simulink model "Test"  (R2021b)
settings: Solver=VariableStepAuto  StartTime=0.0  StopTime=10.0  RelTol=1e-3
undefined symbols (not defined in the file): id, IOSIG_AI_FUEL_IN, NVM_CFG_VEHCLE_MODEL, rte_set_uint8_val, RXSIG_CPD1_FuelMassSignal, SIG_CLASS_COMRX, SIG_CLASS_COMTX, SIG_CLASS_HMI_SND, SIG_CLASS_HMI_TT, SIG_CLASS_IOAL, SIG_CLASS_NVM_CFG, SIG_CLASS_SWC, SIG_CLASS_SYS, SND_FUEL_LEVEL_LOW, SYSSIG_LNN_MODE, SYSSIG_TICK_COUNT, TNC_FuelPrcDisp, TNC_FuelPrcReal, TT_FUEL_LEVEL_LOW, TXSIG_MD_OilPercent, type, val, VEL_VehicleRealSpeed
libraries: simulink x1
(part 1 of 2)
settings Model: Creator=黄艳龙  LastModifiedBy=黄艳龙

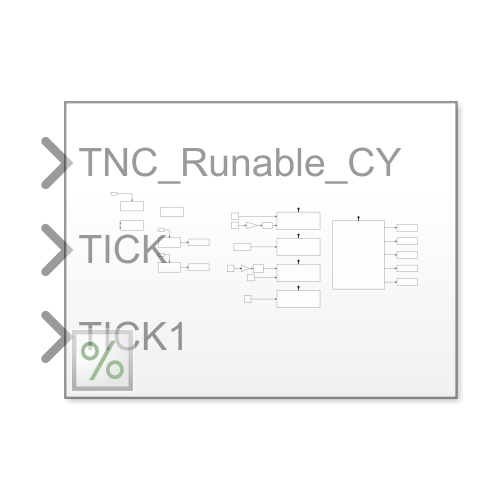
[thumbnail: Simulink's stored preview of the top-level diagram]
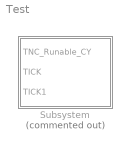
== system Test ==
  Subsystem : Subsystem  Commented=on

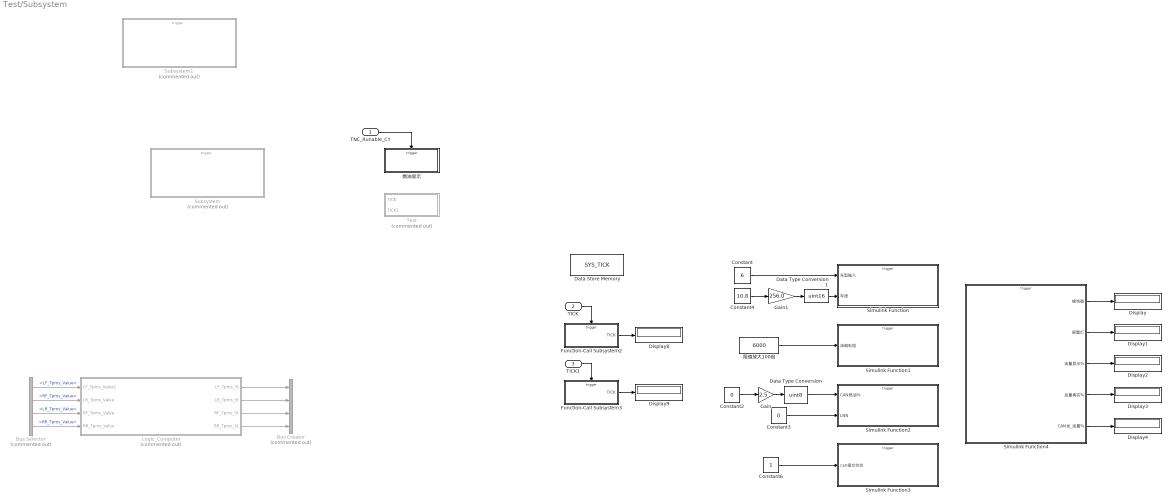
== system Test/Subsystem ==
  TNC_Runable_CY : Inport  SampleTime=1  OutputFunctionCall=on
  TICK : Inport  Priority=1  Port=2  SampleTime=0.001  OutputFunctionCall=on
  TICK1 : Inport  Priority=1  Port=3  SampleTime=0.001  OutputFunctionCall=on
  Bus Creator : BusCreator  Commented=on  Inputs=4
  Bus Selector : BusSelector  Commented=on  OutputSignals=LF_Tpms_Value,RF_Tpms_Value,LR_Tpms_Value,RR_Tpms_Value
  Constant : Constant  Value=6  OutDataTypeStr=uint16
  Constant2 : Constant  Value=0  OutDataTypeStr=single
  Constant3 : Constant  Value=0  OutDataTypeStr=uint8
  Constant4 : Constant  Value=10.8  OutDataTypeStr=single
  Constant6 : Constant  OutDataTypeStr=uint8
  Data Store Memory : DataStoreMemory  DataStoreName=SYS_TICK  ReadBeforeWriteMsg=warning  WriteAfterWriteMsg=warning  WriteAfterReadMsg=warning  ShowAdditionalParam=off  OutDataTypeStr=uint32
  Data Type Conversion : DataTypeConversion  OutDataTypeStr=uint8  RndMeth=Round
  Data Type Conversion1 : DataTypeConversion  OutDataTypeStr=uint16  RndMeth=Round
  Display{,1..4,8..9} (7 alike) : Display
      settings: Format=decimal (Stored Integer)
  Function-Call Subsystem2 : Subsystem  TreatAsAtomicUnit=on
  Function-Call Subsystem3 : Subsystem  TreatAsAtomicUnit=on
  Gain : Gain  Gain=2.5  ParamDataTypeStr=single  OutDataTypeStr=uint8  RndMeth=Round
  Gain1 : Gain  Gain=256.0  ParamDataTypeStr=single  OutDataTypeStr=single
  Logic_Computer : Subsystem  Commented=on
  Simulink Function : Subsystem  TreatAsAtomicUnit=on
  Simulink Function1 : Subsystem  TreatAsAtomicUnit=on
  Simulink Function2 : Subsystem  TreatAsAtomicUnit=on
  Simulink Function3 : Subsystem  TreatAsAtomicUnit=on
  Simulink Function4 : Subsystem  TreatAsAtomicUnit=on
  Subsystem : Subsystem  Commented=on
  Subsystem1 : Subsystem  Commented=on
  Test : Subsystem  Commented=on
  燃油显示 : Subsystem  TreatAsAtomicUnit=on
  阻值放大100倍 : Constant  Value=6000  OutDataTypeStr=uint32
  wires:
  Data Type Conversion1/1 -> Simulink Function/2(车速)
  Constant/1 -> Simulink Function/1(车型输入)
  Gain/1 -> Data Type Conversion/1
  Simulink Function4/1(蜂鸣器) -> Display/1
  Gain1/1 -> Data Type Conversion1/1
  TICK/1 -> Function-Call Subsystem2/Trigger
  Simulink Function4/5(CAN发_油量%) -> Display4/1
  Function-Call Subsystem2/1(TICK) -> Display8/1
  Simulink Function4/3(油量显示%) -> Display2/1
  阻值放大100倍/1 -> Simulink Function1/1(油箱电阻)
  Simulink Function4/4(油量真实%) -> Display3/1
  Data Type Conversion/1 -> Simulink Function2/1(CAN燃油%)
  Constant4/1 -> Gain1/1
  Constant6/1 -> Simulink Function3/1(can报文状态)
  Simulink Function4/2(报警灯) -> Display1/1
  Constant3/1 -> Simulink Function2/2(LNN)
  TICK1/1 -> Function-Call Subsystem3/Trigger
  Function-Call Subsystem3/1(TICK) -> Display9/1
  Constant2/1 -> Gain/1
  TNC_Runable_CY/1 -> 燃油显示/Trigger
  Bus Selector/3 -> Logic_Computer/3(RF_Tpms_Value)  "<LR_Tpms_Value>"
  Logic_Computer/1(LF_Tpms_St) -> Bus Creator/1
  Logic_Computer/2(LR_Tpms_St) -> Bus Creator/2
  Bus Selector/2 -> Logic_Computer/2(LR_Tpms_Value)  "<RF_Tpms_Value>"
  Bus Selector/4 -> Logic_Computer/4(RR_Tpms_Value)  "<RR_Tpms_Value>"
  Bus Selector/1 -> Logic_Computer/1(LF_Tpms_Value1)  "<LF_Tpms_Value>"
  Logic_Computer/3(RF_Tpms_St) -> Bus Creator/3
  Logic_Computer/4(RR_Tpms_St) -> Bus Creator/4

== system Test/Subsystem/Function-Call Subsystem2 ==
  function : TriggerPort  TriggerType=function-call  VariantControl=(inherit)
  Add : Sum
  Constant : Constant  OutDataTypeStr=uint32
  Data Store Read : DataStoreRead  DataStoreName=SYS_TICK  IndexOptions=Index vector (dialog)  Indices=1  OutputSizes=1
  Data Store Write : DataStoreWrite  DataStoreName=SYS_TICK  IndexOptions=Index vector (dialog)  Indices=1  OutputSizes=1
  TICK : Outport  OutDataTypeStr=uint32
  wires:
  Data Store Read/1 -> Add/1
  Add/1 -> TICK/1, Data Store Write/1
  Constant/1 -> Add/2

== system Test/Subsystem/Function-Call Subsystem3 ==
  function : TriggerPort  TriggerType=function-call  VariantControl=(inherit)
  Add : Sum
  Constant : Constant  OutDataTypeStr=uint32
  Data Store Write : DataStoreWrite  Commented=on  DataStoreName=SYS_TICK  IndexOptions=Index vector (dialog)  Indices=1  OutputSizes=1
  Unit Delay : UnitDelay  SampleTime=-1  HasFrameUpgradeWarning=on
  TICK : Outport  OutDataTypeStr=uint32
  wires:
  Add/1 -> Data Store Write/1, Unit Delay/1, TICK/1
  Constant/1 -> Add/1
  Unit Delay/1 -> Add/2

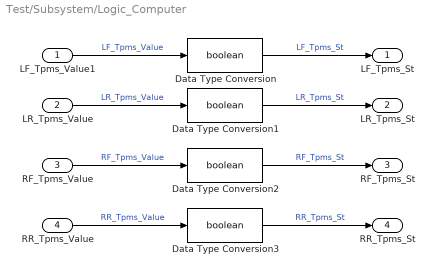
== system Test/Subsystem/Logic_Computer ==
  LF_Tpms_Value1 : Inport
  LR_Tpms_Value : Inport  Port=2
  RF_Tpms_Value : Inport  Port=3
  RR_Tpms_Value : Inport  Port=4
  Data Type Conversion{,1..3} (4 alike) : DataTypeConversion  OutDataTypeStr=boolean
  LF_Tpms_St : Outport
  LR_Tpms_St : Outport  Port=2
  RF_Tpms_St : Outport  Port=3
  RR_Tpms_St : Outport  Port=4
  wires:
  RR_Tpms_Value/1 -> Data Type Conversion3/1  "RR_Tpms_Value"
  RF_Tpms_Value/1 -> Data Type Conversion2/1  "RF_Tpms_Value"
  LR_Tpms_Value/1 -> Data Type Conversion1/1  "LR_Tpms_Value"
  LF_Tpms_Value1/1 -> Data Type Conversion/1  "LF_Tpms_Value"
  Data Type Conversion/1 -> LF_Tpms_St/1  "LF_Tpms_St"
  Data Type Conversion1/1 -> LR_Tpms_St/1  "LR_Tpms_St"
  Data Type Conversion2/1 -> RF_Tpms_St/1  "RF_Tpms_St"
  Data Type Conversion3/1 -> RR_Tpms_St/1  "RR_Tpms_St"

== system Test/Subsystem/Simulink Function ==
  车型输入 : Inport  OutDataTypeStr=uint16
  车速 : Inport  Port=2  OutDataTypeStr=uint16
  rte_get_uint16_val : TriggerPort  TriggerType=function-call  IsSimulinkFunction=on  FunctionName=rte_get_uint16_val  FunctionVisibility=scoped  VariantControl=(inherit)
  If : If  IfExpression=u1==21  ElseIfExpressions=u1==18  ShowElse=off
  Merge : Merge
  Terminator : Terminator
  车型_ : Subsystem  TreatAsAtomicUnit=on
  车速_ : Subsystem  TreatAsAtomicUnit=on
  type : ArgIn  DisableCoverage=on  OutDataTypeStr=uint8  ArgumentName=type
  id : ArgIn  DisableCoverage=on  Port=2  OutDataTypeStr=uint16  ArgumentName=id
  val : ArgOut  DisableCoverage=on  OutDataTypeStr=uint16  ArgumentName=val
  wires:
  type/1 -> Terminator/1
  id/1 -> If/1
  If/1 -> 车型_/Action
  If/2 -> 车速_/Action
  车型_/1(Out1) -> Merge/1
  车速_/1(Out1) -> Merge/2
  Merge/1 -> val/1
  车型输入/1 -> 车型_/1(车型输入)
  车速/1 -> 车速_/1(车型输入1)

== system Test/Subsystem/Simulink Function1 ==
  油箱电阻 : Inport  OutDataTypeStr=uint32
  rte_get_uint32_val : TriggerPort  TriggerType=function-call  IsSimulinkFunction=on  FunctionName=rte_get_uint32_val  FunctionVisibility=scoped  VariantControl=(inherit)
  Data Store Read : DataStoreRead  DataStoreName=SYS_TICK  IndexOptions=Index vector (dialog)  Indices=1  OutputSizes=1
  If : If  IfExpression=u1==17  ElseIfExpressions=u1==14  ShowElse=off
  If Action Subsystem : Subsystem  TreatAsAtomicUnit=on
  If Action Subsystem1 : Subsystem  TreatAsAtomicUnit=on
  Merge : Merge
  Terminator : Terminator
  type : ArgIn  DisableCoverage=on  OutDataTypeStr=uint8  ArgumentName=type
  id : ArgIn  DisableCoverage=on  Port=2  OutDataTypeStr=uint16  ArgumentName=id
  val : ArgOut  DisableCoverage=on  OutDataTypeStr=uint32  ArgumentName=val
  wires:
  type/1 -> Terminator/1
  id/1 -> If/1
  Merge/1 -> val/1
  If/1 -> If Action Subsystem/Action
  油箱电阻/1 -> If Action Subsystem/1(油箱电阻)
  Data Store Read/1 -> If Action Subsystem1/1(时间)
  If/2 -> If Action Subsystem1/Action
  If Action Subsystem/1(Out1) -> Merge/1
  If Action Subsystem1/1(Out1) -> Merge/2

== system Test/Subsystem/Simulink Function2 ==
  CAN燃油% : Inport  OutDataTypeStr=uint8
  LNN : Inport  Port=2  OutDataTypeStr=uint8
  rte_get_uint8_val : TriggerPort  TriggerType=function-call  IsSimulinkFunction=on  FunctionName=rte_get_uint8_val  FunctionVisibility=scoped  VariantControl=(inherit)
  Merge : Merge
  Switch Case : SwitchCase  CaseConditions={15,13}
  Terminator : Terminator
  Terminator1 : Terminator
  _ : Subsystem  TreatAsAtomicUnit=on
  车速_ : Subsystem  TreatAsAtomicUnit=on
  u : ArgIn  DisableCoverage=on  OutDataTypeStr=uint8  ArgumentName=type
  u1 : ArgIn  DisableCoverage=on  Port=2  OutDataTypeStr=uint16  ArgumentName=id
  y : ArgOut  DisableCoverage=on  OutDataTypeStr=uint8  ArgumentName=val
  wires:
  u/1 -> Terminator/1
  u1/1 -> Switch Case/1
  Switch Case/1 -> _/Action
  _/1(Out1) -> Merge/1
  车速_/1(Out1) -> Merge/2
  Merge/1 -> y/1
  CAN燃油%/1 -> _/1(in)
  LNN/1 -> 车速_/1(in)
  Switch Case/2 -> 车速_/Action
  Switch Case/3 -> Terminator1/1

== system Test/Subsystem/Simulink Function3 ==
  can报文状态 : Inport  OutDataTypeStr=uint8
  rte_com_get_rxsig_state : TriggerPort  TriggerType=function-call  IsSimulinkFunction=on  FunctionName=rte_com_get_rxsig_state  FunctionVisibility=scoped  VariantControl=(inherit)
  Terminator1 : Terminator
  id : ArgIn  DisableCoverage=on  OutDataTypeStr=uint16  ArgumentName=id
  val : ArgOut  DisableCoverage=on  OutDataTypeStr=uint8  ArgumentName=val
  wires:
  id/1 -> Terminator1/1
  can报文状态/1 -> val/1

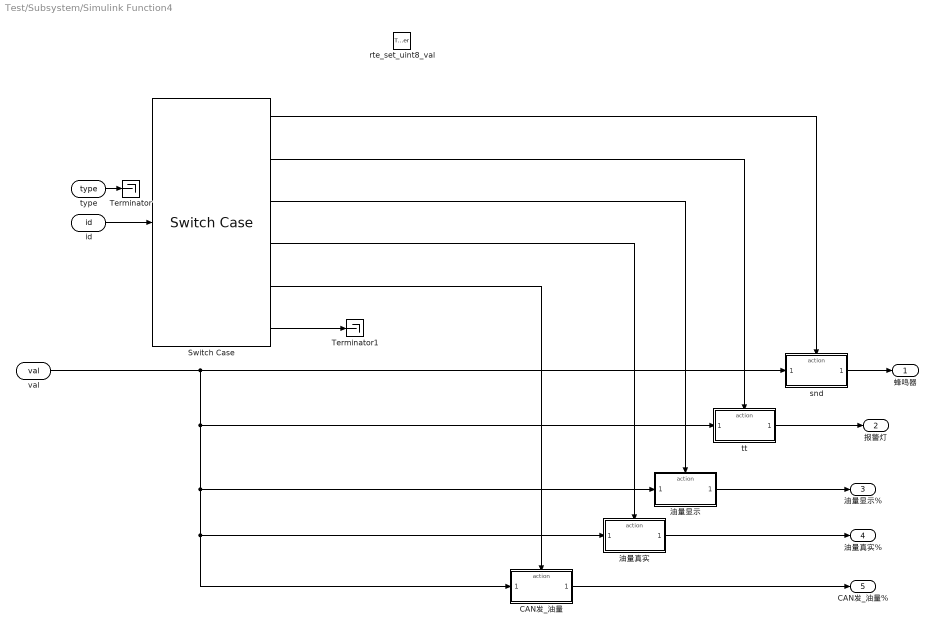
== system Test/Subsystem/Simulink Function4 ==
  rte_set_uint8_val : TriggerPort  TriggerType=function-call  IsSimulinkFunction=on  FunctionName=rte_set_uint8_val  FunctionVisibility=scoped  VariantControl=(inherit)
  CAN发_油量 : Subsystem  TreatAsAtomicUnit=on
  Switch Case : SwitchCase  CaseConditions={23,22,19,20,16}
  Terminator : Terminator
  Terminator1 : Terminator
  snd : Subsystem  TreatAsAtomicUnit=on
  tt : Subsystem  TreatAsAtomicUnit=on
  油量显示 : Subsystem  TreatAsAtomicUnit=on
  油量真实 : Subsystem  TreatAsAtomicUnit=on
  type : ArgIn  DisableCoverage=on  OutDataTypeStr=uint8  ArgumentName=type
  id : ArgIn  DisableCoverage=on  Port=2  OutDataTypeStr=uint16  ArgumentName=id
  val : ArgIn  DisableCoverage=on  Port=3  OutDataTypeStr=uint8  ArgumentName=val
  蜂鸣器 : Outport  OutDataTypeStr=uint8
  报警灯 : Outport  Port=2  OutDataTypeStr=uint8
  油量显示% : Outport  Port=3  OutDataTypeStr=uint8
  油量真实% : Outport  Port=4  OutDataTypeStr=uint8
  CAN发_油量% : Outport  Port=5  OutDataTypeStr=uint8
  wires:
  type/1 -> Terminator/1
  id/1 -> Switch Case/1
  snd/1(Output) -> 蜂鸣器/1
  tt/1(Output1) -> 报警灯/1
  Switch Case/1 -> snd/Action
  Switch Case/2 -> tt/Action
  Switch Case/3 -> 油量显示/Action
  油量显示/1(Output1) -> 油量显示%/1
  Switch Case/4 -> 油量真实/Action
  油量真实/1(Output1) -> 油量真实%/1
  Switch Case/5 -> CAN发_油量/Action
  CAN发_油量/1(Output1) -> CAN发_油量%/1
  val/1 -> snd/1(车型输入), tt/1(车型输入), CAN发_油量/1(车型输入), 油量真实/1(车型输入), 油量显示/1(车型输入)
  Switch Case/6 -> Terminator1/1

== system Test/Subsystem/Subsystem ==
  function : TriggerPort  TriggerType=function-call  VariantControl=(inherit)
  Constant : Constant
  Constant1 : Constant
  Function Caller : FunctionCaller  FunctionPrototype=val = rte_get_uint8_val(x,y)  InputArgumentSpecifications=<Enter example>  OutputArgumentSpecifications=<Enter example>
  Scope : Scope
  Simulink Function : Subsystem  TreatAsAtomicUnit=on
  wires:
  Constant/1 -> Function Caller/1
  Constant1/1 -> Function Caller/2
  Function Caller/1 -> Scope/1

== system Test/Subsystem/Subsystem1 ==
  function : TriggerPort  TriggerType=function-call  VariantControl=(inherit)
  Constant : Constant
  Constant1 : Constant
  Function Caller : FunctionCaller  FunctionPrototype=val = rte_get_uint8_val(x,y)  InputArgumentSpecifications=<Enter example>  OutputArgumentSpecifications=<Enter example>
  Scope : Scope
  Simulink Function : Subsystem  TreatAsAtomicUnit=on
  wires:
  Constant/1 -> Function Caller/1
  Constant1/1 -> Function Caller/2
  Function Caller/1 -> Scope/1

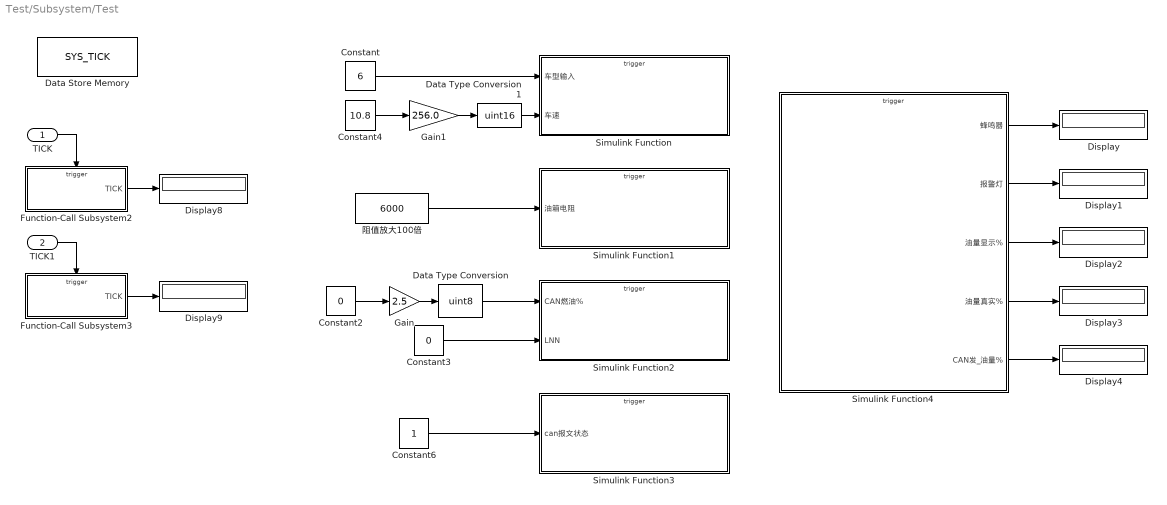
== system Test/Subsystem/Test ==
  TICK : Inport  Priority=1  SampleTime=0.001  OutputFunctionCall=on
  TICK1 : Inport  Priority=1  Port=2  SampleTime=0.001  OutputFunctionCall=on
  Constant : Constant  Value=6  OutDataTypeStr=uint16
  Constant2 : Constant  Value=0  OutDataTypeStr=single
  Constant3 : Constant  Value=0  OutDataTypeStr=uint8
  Constant4 : Constant  Value=10.8  OutDataTypeStr=single
  Constant6 : Constant  OutDataTypeStr=uint8
  Data Store Memory : DataStoreMemory  DataStoreName=SYS_TICK  ReadBeforeWriteMsg=warning  WriteAfterWriteMsg=warning  WriteAfterReadMsg=warning  ShowAdditionalParam=off  OutDataTypeStr=uint32
  Data Type Conversion : DataTypeConversion  OutDataTypeStr=uint8  RndMeth=Round
  Data Type Conversion1 : DataTypeConversion  OutDataTypeStr=uint16  RndMeth=Round
  Display{,1..4,8..9} (7 alike) : Display
      settings: Format=decimal (Stored Integer)
  Function-Call Subsystem2 : Subsystem  TreatAsAtomicUnit=on
  Function-Call Subsystem3 : Subsystem  TreatAsAtomicUnit=on
  Gain : Gain  Gain=2.5  ParamDataTypeStr=single  OutDataTypeStr=uint8  RndMeth=Round
  Gain1 : Gain  Gain=256.0  ParamDataTypeStr=single  OutDataTypeStr=single
  Simulink Function : Subsystem  TreatAsAtomicUnit=on
  Simulink Function1 : Subsystem  TreatAsAtomicUnit=on
  Simulink Function2 : Subsystem  TreatAsAtomicUnit=on
  Simulink Function3 : Subsystem  TreatAsAtomicUnit=on
  Simulink Function4 : Subsystem  TreatAsAtomicUnit=on
  阻值放大100倍 : Constant  Value=6000  OutDataTypeStr=uint32
  wires:
  Constant/1 -> Simulink Function/1(车型输入)
  Simulink Function4/3(油量显示%) -> Display2/1
  Simulink Function4/2(报警灯) -> Display1/1
  Function-Call Subsystem3/1(TICK) -> Display9/1
  Simulink Function4/5(CAN发_油量%) -> Display4/1
  Constant4/1 -> Gain1/1
  Simulink Function4/4(油量真实%) -> Display3/1
  Constant6/1 -> Simulink Function3/1(can报文状态)
  Constant3/1 -> Simulink Function2/2(LNN)
  Constant2/1 -> Gain/1
  Gain/1 -> Data Type Conversion/1
  TICK/1 -> Function-Call Subsystem2/Trigger
  Function-Call Subsystem2/1(TICK) -> Display8/1
  阻值放大100倍/1 -> Simulink Function1/1(油箱电阻)
  Data Type Conversion1/1 -> Simulink Function/2(车速)
  Gain1/1 -> Data Type Conversion1/1
  TICK1/1 -> Function-Call Subsystem3/Trigger
  Simulink Function4/1(蜂鸣器) -> Display/1
  Data Type Conversion/1 -> Simulink Function2/1(CAN燃油%)

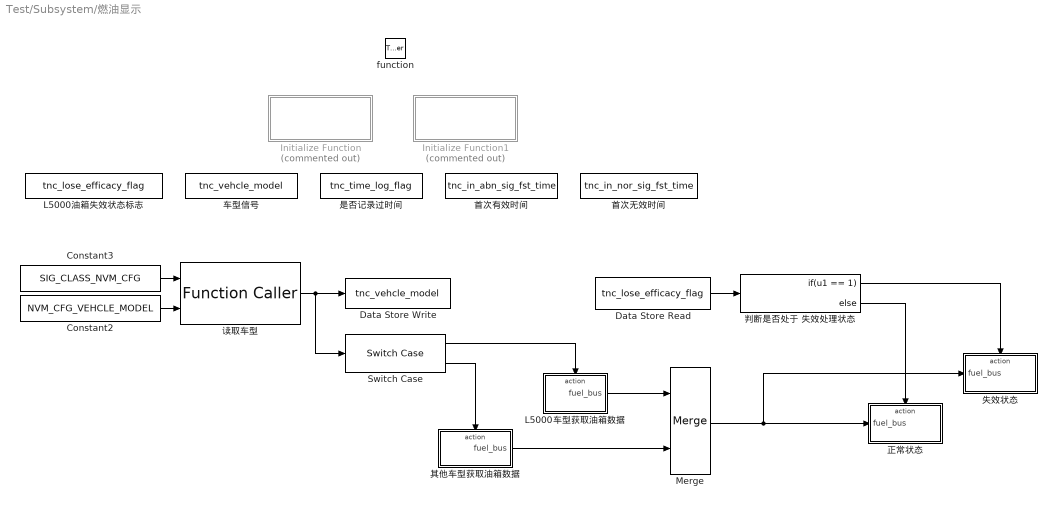
== system Test/Subsystem/燃油显示 ==
  function : TriggerPort  TriggerType=function-call  VariantControl=(inherit)
  Constant2 : Constant  Value=NVM_CFG_VEHCLE_MODEL  OutDataTypeStr=uint16
  Constant3 : Constant  Value=SIG_CLASS_NVM_CFG  OutDataTypeStr=uint8
  Data Store Read : DataStoreRead  DataStoreName=tnc_lose_efficacy_flag  IndexOptions=Index vector (dialog)  Indices=1  OutputSizes=1
  Data Store Write : DataStoreWrite  DataStoreName=tnc_vehcle_model  IndexOptions=Index vector (dialog)  Indices=1  OutputSizes=1
  Initialize Function : Subsystem  Priority=0  Commented=on  TreatAsAtomicUnit=on
  Initialize Function1 : Subsystem  Commented=on  TreatAsAtomicUnit=on
  L5000油箱失效状态标志 : DataStoreMemory  DataStoreName=tnc_lose_efficacy_flag  ReadBeforeWriteMsg=warning  WriteAfterWriteMsg=warning  WriteAfterReadMsg=warning  ShowAdditionalParam=off  OutDataTypeStr=uint8  StateMustResolveToSignalObject=on
  L5000车型获取油箱数据 : Subsystem  TreatAsAtomicUnit=on
  Merge : Merge
  Switch Case : SwitchCase  CaseConditions={[6]}
  其他车型获取油箱数据 : Subsystem  TreatAsAtomicUnit=on
  判断是否处于 失效处理状态 : If  IfExpression=u1 == 1
  失效状态 : Subsystem  TreatAsAtomicUnit=on
  是否记录过时间 : DataStoreMemory  DataStoreName=tnc_time_log_flag  ReadBeforeWriteMsg=warning  WriteAfterWriteMsg=warning  WriteAfterReadMsg=warning  ShowAdditionalParam=off  OutDataTypeStr=uint8  StateMustResolveToSignalObject=on
  正常状态 : Subsystem  TreatAsAtomicUnit=on
  读取车型 : FunctionCaller  FunctionPrototype=val = rte_get_uint16_val(type,id)  InputArgumentSpecifications=uint8(1),uint16(1)  OutputArgumentSpecifications=uint16(1)
  车型信号 : DataStoreMemory  Priority=1  DataStoreName=tnc_vehcle_model  ReadBeforeWriteMsg=warning  WriteAfterWriteMsg=warning  WriteAfterReadMsg=warning  ShowAdditionalParam=off  OutDataTypeStr=uint16
  首次无效时间 : DataStoreMemory  DataStoreName=tnc_in_nor_sig_fst_time  ReadBeforeWriteMsg=warning  WriteAfterWriteMsg=warning  WriteAfterReadMsg=warning  ShowAdditionalParam=off  OutDataTypeStr=uint32  StateMustResolveToSignalObject=on
  首次有效时间 : DataStoreMemory  DataStoreName=tnc_in_abn_sig_fst_time  ReadBeforeWriteMsg=warning  WriteAfterWriteMsg=warning  WriteAfterReadMsg=warning  ShowAdditionalParam=off  OutDataTypeStr=uint32  StateMustResolveToSignalObject=on
  wires:
  L5000车型获取油箱数据/1(fuel_bus) -> Merge/1
  读取车型/1 -> Switch Case/1, Data Store Write/1
  Data Store Read/1 -> 判断是否处于 失效处理状态/1
  判断是否处于 失效处理状态/1 -> 失效状态/Action
  Merge/1 -> 失效状态/1(fuel_bus), 正常状态/1(fuel_bus)
  其他车型获取油箱数据/1(fuel_bus) -> Merge/2
  Constant3/1 -> 读取车型/1
  判断是否处于 失效处理状态/2 -> 正常状态/Action
  Switch Case/1 -> L5000车型获取油箱数据/Action
  Switch Case/2 -> 其他车型获取油箱数据/Action
  Constant2/1 -> 读取车型/2

== system Test/Subsystem/Simulink Function/车型_ ==
  车型输入 : Inport  OutDataTypeStr=uint16
  Action Port : ActionPort
  Out1 : Outport  OutDataTypeStr=uint16
  wires:
  车型输入/1 -> Out1/1

== system Test/Subsystem/Simulink Function/车速_ ==
  车型输入1 : Inport  OutDataTypeStr=uint16
  Action Port : ActionPort
  Out1 : Outport  OutDataTypeStr=uint16
  wires:
  车型输入1/1 -> Out1/1

== system Test/Subsystem/Simulink Function1/If Action Subsystem ==
  油箱电阻 : Inport  OutDataTypeStr=uint32
  Action Port : ActionPort
  Out1 : Outport  OutDataTypeStr=uint32
  wires:
  油箱电阻/1 -> Out1/1

== system Test/Subsystem/Simulink Function1/If Action Subsystem1 ==
  时间 : Inport  OutDataTypeStr=uint32
  Action Port : ActionPort
  Out1 : Outport  OutDataTypeStr=uint32
  wires:
  时间/1 -> Out1/1

== system Test/Subsystem/Simulink Function2/_ ==
  in : Inport  OutDataTypeStr=uint8
  Action Port : ActionPort
  Out1 : Outport  OutDataTypeStr=uint8
  wires:
  in/1 -> Out1/1

== system Test/Subsystem/Simulink Function2/车速_ ==
  in : Inport  OutDataTypeStr=uint8
  Action Port : ActionPort
  Out1 : Outport  OutDataTypeStr=uint8
  wires:
  in/1 -> Out1/1

== system Test/Subsystem/Simulink Function4/CAN发_油量 ==
  车型输入 : Inport  OutDataTypeStr=uint8
  Action Port : ActionPort
  Output1 : Outport  OutDataTypeStr=uint8
  wires:
  车型输入/1 -> Output1/1

== system Test/Subsystem/Simulink Function4/snd ==
  车型输入 : Inport  OutDataTypeStr=uint8
  Action Port : ActionPort
  Output : Outport  OutDataTypeStr=uint8
  wires:
  车型输入/1 -> Output/1

== system Test/Subsystem/Simulink Function4/tt ==
  车型输入 : Inport  OutDataTypeStr=uint8
  Action Port : ActionPort
  Output1 : Outport  OutDataTypeStr=uint8
  wires:
  车型输入/1 -> Output1/1

== system Test/Subsystem/Simulink Function4/油量显示 ==
  车型输入 : Inport  OutDataTypeStr=uint8
  Action Port : ActionPort
  Output1 : Outport  OutDataTypeStr=uint8
  wires:
  车型输入/1 -> Output1/1

== system Test/Subsystem/Simulink Function4/油量真实 ==
  车型输入 : Inport  OutDataTypeStr=uint8
  Action Port : ActionPort
  Output1 : Outport  OutDataTypeStr=uint8
  wires:
  车型输入/1 -> Output1/1

== system Test/Subsystem/Subsystem/Simulink Function ==
  rte_get_uint8_val : TriggerPort  TriggerType=function-call  IsSimulinkFunction=on  FunctionName=rte_get_uint8_val  FunctionVisibility=scoped  VariantControl=(inherit)
  Constant : Constant
  Gain : Gain  Gain=10
  Sum : Sum  Inputs=|+++
  x : ArgIn  DisableCoverage=on  ArgumentName=x
  y : ArgIn  Port=2  ArgumentName=y
  val : ArgOut  DisableCoverage=on  ArgumentName=val
  wires:
  y/1 -> Sum/2
  Gain/1 -> val/1
  x/1 -> Sum/1
  Constant/1 -> Sum/3
  Sum/1 -> Gain/1

== system Test/Subsystem/Subsystem1/Simulink Function ==
  rte_get_uint8_val : TriggerPort  TriggerType=function-call  IsSimulinkFunction=on  FunctionName=rte_get_uint8_val  FunctionVisibility=scoped  VariantControl=(inherit)
  Constant : Constant
  Gain : Gain  Gain=10
  Sum : Sum  Inputs=|+++
  x : ArgIn  DisableCoverage=on  ArgumentName=x
  y : ArgIn  Port=2  ArgumentName=y
  val : ArgOut  DisableCoverage=on  ArgumentName=val
  wires:
  y/1 -> Sum/2
  Gain/1 -> val/1
  x/1 -> Sum/1
  Constant/1 -> Sum/3
  Sum/1 -> Gain/1

== system Test/Subsystem/Test/Function-Call Subsystem2 ==
  function : TriggerPort  TriggerType=function-call  VariantControl=(inherit)
  Add : Sum
  Constant : Constant  OutDataTypeStr=uint32
  Data Store Read : DataStoreRead  DataStoreName=SYS_TICK  IndexOptions=Index vector (dialog)  Indices=1  OutputSizes=1
  Data Store Write : DataStoreWrite  DataStoreName=SYS_TICK  IndexOptions=Index vector (dialog)  Indices=1  OutputSizes=1
  TICK : Outport  OutDataTypeStr=uint32
  wires:
  Data Store Read/1 -> Add/1
  Add/1 -> TICK/1, Data Store Write/1
  Constant/1 -> Add/2

== system Test/Subsystem/Test/Function-Call Subsystem3 ==
  function : TriggerPort  TriggerType=function-call  VariantControl=(inherit)
  Add : Sum
  Constant : Constant  OutDataTypeStr=uint32
  Data Store Write : DataStoreWrite  Commented=on  DataStoreName=SYS_TICK  IndexOptions=Index vector (dialog)  Indices=1  OutputSizes=1
  Unit Delay : UnitDelay  SampleTime=-1  HasFrameUpgradeWarning=on
  TICK : Outport  OutDataTypeStr=uint32
  wires:
  Add/1 -> Data Store Write/1, Unit Delay/1, TICK/1
  Constant/1 -> Add/1
  Unit Delay/1 -> Add/2

== system Test/Subsystem/Test/Simulink Function ==
  车型输入 : Inport  OutDataTypeStr=uint16
  车速 : Inport  Port=2  OutDataTypeStr=uint16
  rte_get_uint16_val : TriggerPort  TriggerType=function-call  IsSimulinkFunction=on  FunctionName=rte_get_uint16_val  FunctionVisibility=scoped  VariantControl=(inherit)
  If : If  IfExpression=u1==21  ElseIfExpressions=u1==18  ShowElse=off
  Merge : Merge
  Terminator : Terminator
  车型_ : Subsystem  TreatAsAtomicUnit=on
  车速_ : Subsystem  TreatAsAtomicUnit=on
  type : ArgIn  DisableCoverage=on  OutDataTypeStr=uint8  ArgumentName=type
  id : ArgIn  DisableCoverage=on  Port=2  OutDataTypeStr=uint16  ArgumentName=id
  val : ArgOut  DisableCoverage=on  OutDataTypeStr=uint16  ArgumentName=val
  wires:
  type/1 -> Terminator/1
  id/1 -> If/1
  If/1 -> 车型_/Action
  If/2 -> 车速_/Action
  车型_/1(Out1) -> Merge/1
  车速_/1(Out1) -> Merge/2
  Merge/1 -> val/1
  车型输入/1 -> 车型_/1(车型输入)
  车速/1 -> 车速_/1(车型输入1)

== system Test/Subsystem/Test/Simulink Function1 ==
  油箱电阻 : Inport  OutDataTypeStr=uint32
  rte_get_uint32_val : TriggerPort  TriggerType=function-call  IsSimulinkFunction=on  FunctionName=rte_get_uint32_val  FunctionVisibility=scoped  VariantControl=(inherit)
  Data Store Read : DataStoreRead  DataStoreName=SYS_TICK  IndexOptions=Index vector (dialog)  Indices=1  OutputSizes=1
  If : If  IfExpression=u1==17  ElseIfExpressions=u1==14  ShowElse=off
  If Action Subsystem : Subsystem  TreatAsAtomicUnit=on
  If Action Subsystem1 : Subsystem  TreatAsAtomicUnit=on
  Merge : Merge
  Terminator : Terminator
  type : ArgIn  DisableCoverage=on  OutDataTypeStr=uint8  ArgumentName=type
  id : ArgIn  DisableCoverage=on  Port=2  OutDataTypeStr=uint16  ArgumentName=id
  val : ArgOut  DisableCoverage=on  OutDataTypeStr=uint32  ArgumentName=val
  wires:
  type/1 -> Terminator/1
  id/1 -> If/1
  Merge/1 -> val/1
  If/1 -> If Action Subsystem/Action
  油箱电阻/1 -> If Action Subsystem/1(油箱电阻)
  Data Store Read/1 -> If Action Subsystem1/1(时间)
  If/2 -> If Action Subsystem1/Action
  If Action Subsystem/1(Out1) -> Merge/1
  If Action Subsystem1/1(Out1) -> Merge/2

== system Test/Subsystem/Test/Simulink Function2 ==
  CAN燃油% : Inport  OutDataTypeStr=uint8
  LNN : Inport  Port=2  OutDataTypeStr=uint8
  rte_get_uint8_val : TriggerPort  TriggerType=function-call  IsSimulinkFunction=on  FunctionName=rte_get_uint8_val  FunctionVisibility=scoped  VariantControl=(inherit)
  Merge : Merge
  Switch Case : SwitchCase  CaseConditions={15,13}
  Terminator : Terminator
  Terminator1 : Terminator
  _ : Subsystem  TreatAsAtomicUnit=on
  车速_ : Subsystem  TreatAsAtomicUnit=on
  u : ArgIn  DisableCoverage=on  OutDataTypeStr=uint8  ArgumentName=type
  u1 : ArgIn  DisableCoverage=on  Port=2  OutDataTypeStr=uint16  ArgumentName=id
  y : ArgOut  DisableCoverage=on  OutDataTypeStr=uint8  ArgumentName=val
  wires:
  u/1 -> Terminator/1
  u1/1 -> Switch Case/1
  Switch Case/1 -> _/Action
  _/1(Out1) -> Merge/1
  车速_/1(Out1) -> Merge/2
  Merge/1 -> y/1
  CAN燃油%/1 -> _/1(in)
  LNN/1 -> 车速_/1(in)
  Switch Case/2 -> 车速_/Action
  Switch Case/3 -> Terminator1/1

== system Test/Subsystem/Test/Simulink Function3 ==
  can报文状态 : Inport  OutDataTypeStr=uint8
  rte_com_get_rxsig_state : TriggerPort  TriggerType=function-call  IsSimulinkFunction=on  FunctionName=rte_com_get_rxsig_state  FunctionVisibility=scoped  VariantControl=(inherit)
  Terminator1 : Terminator
  id : ArgIn  DisableCoverage=on  OutDataTypeStr=uint16  ArgumentName=id
  val : ArgOut  DisableCoverage=on  OutDataTypeStr=uint8  ArgumentName=val
  wires:
  id/1 -> Terminator1/1
  can报文状态/1 -> val/1

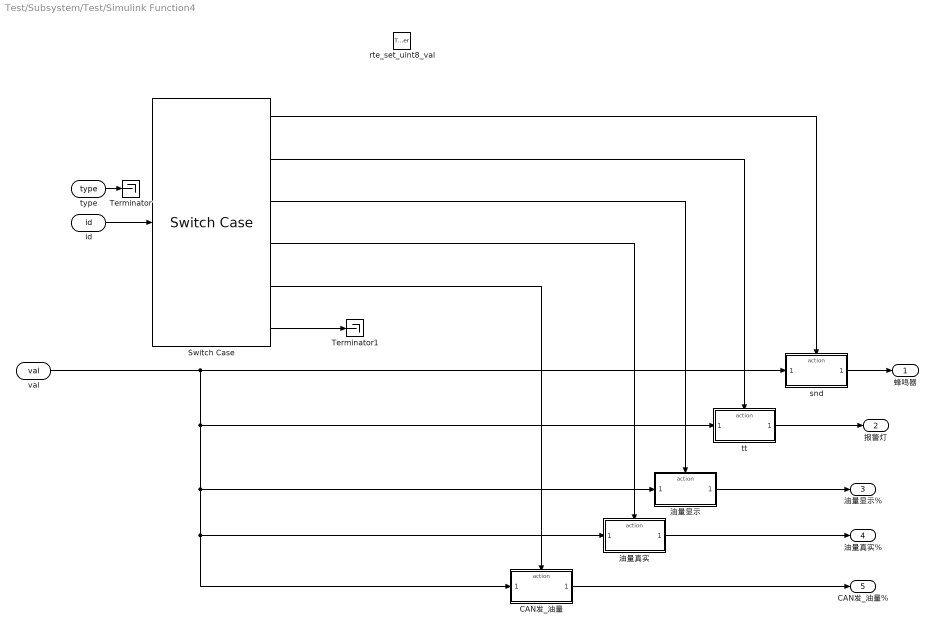
== system Test/Subsystem/Test/Simulink Function4 ==
  rte_set_uint8_val : TriggerPort  TriggerType=function-call  IsSimulinkFunction=on  FunctionName=rte_set_uint8_val  FunctionVisibility=scoped  VariantControl=(inherit)
  CAN发_油量 : Subsystem  TreatAsAtomicUnit=on
  Switch Case : SwitchCase  CaseConditions={23,22,19,20,16}
  Terminator : Terminator
  Terminator1 : Terminator
  snd : Subsystem  TreatAsAtomicUnit=on
  tt : Subsystem  TreatAsAtomicUnit=on
  油量显示 : Subsystem  TreatAsAtomicUnit=on
  油量真实 : Subsystem  TreatAsAtomicUnit=on
  type : ArgIn  DisableCoverage=on  OutDataTypeStr=uint8  ArgumentName=type
  id : ArgIn  DisableCoverage=on  Port=2  OutDataTypeStr=uint16  ArgumentName=id
  val : ArgIn  DisableCoverage=on  Port=3  OutDataTypeStr=uint8  ArgumentName=val
  蜂鸣器 : Outport  OutDataTypeStr=uint8
  报警灯 : Outport  Port=2  OutDataTypeStr=uint8
  油量显示% : Outport  Port=3  OutDataTypeStr=uint8
  油量真实% : Outport  Port=4  OutDataTypeStr=uint8
  CAN发_油量% : Outport  Port=5  OutDataTypeStr=uint8
  wires:
  type/1 -> Terminator/1
  id/1 -> Switch Case/1
  snd/1(Output) -> 蜂鸣器/1
  tt/1(Output1) -> 报警灯/1
  Switch Case/1 -> snd/Action
  Switch Case/2 -> tt/Action
  Switch Case/3 -> 油量显示/Action
  油量显示/1(Output1) -> 油量显示%/1
  Switch Case/4 -> 油量真实/Action
  油量真实/1(Output1) -> 油量真实%/1
  Switch Case/5 -> CAN发_油量/Action
  CAN发_油量/1(Output1) -> CAN发_油量%/1
  val/1 -> snd/1(车型输入), tt/1(车型输入), CAN发_油量/1(车型输入), 油量真实/1(车型输入), 油量显示/1(车型输入)
  Switch Case/6 -> Terminator1/1

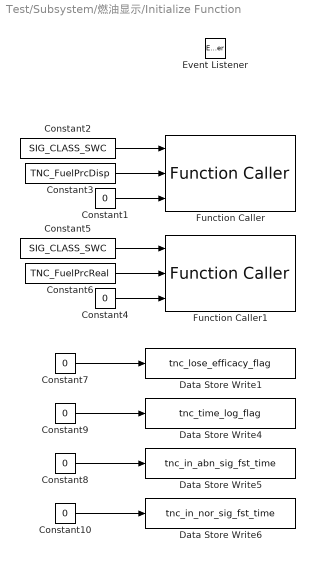
== system Test/Subsystem/燃油显示/Initialize Function ==
  Constant{1,4,7,9} (4 alike) : Constant  Value=0  OutDataTypeStr=uint8
  Constant10 : Constant  Value=0  OutDataTypeStr=uint32
  Constant2 : Constant  Value=SIG_CLASS_SWC  OutDataTypeStr=uint8
  Constant3 : Constant  Value=TNC_FuelPrcDisp  OutDataTypeStr=uint16
  Constant5 : Constant  Value=SIG_CLASS_SWC  OutDataTypeStr=uint8
  Constant6 : Constant  Value=TNC_FuelPrcReal  OutDataTypeStr=uint16
  Constant8 : Constant  Value=0  OutDataTypeStr=uint32
  Data Store Write1 : DataStoreWrite  DataStoreName=tnc_lose_efficacy_flag  IndexOptions=Index vector (dialog)  Indices=1  OutputSizes=1
  Data Store Write4 : DataStoreWrite  DataStoreName=tnc_time_log_flag  IndexOptions=Index vector (dialog)  Indices=1  OutputSizes=1
  Data Store Write5 : DataStoreWrite  DataStoreName=tnc_in_abn_sig_fst_time  IndexOptions=Index vector (dialog)  Indices=1  OutputSizes=1
  Data Store Write6 : DataStoreWrite  DataStoreName=tnc_in_nor_sig_fst_time  IndexOptions=Index vector (dialog)  Indices=1  OutputSizes=1
  Event Listener : EventListener  DisableCoverage=on  EventName=reset
  Function Caller : FunctionCaller  FunctionPrototype=rte_set_uint8_val(type,id,val)  InputArgumentSpecifications=uint8(1), uint16(1), uint8(1)  OutputArgumentSpecifications=<Enter example>
  Function Caller1 : FunctionCaller  FunctionPrototype=rte_set_uint8_val(type,id,val)  InputArgumentSpecifications=uint8(1), uint16(1), uint8(1)  OutputArgumentSpecifications=<Enter example>
  wires:
  Constant5/1 -> Function Caller1/1
  Constant3/1 -> Function Caller/2
  Constant1/1 -> Function Caller/3
  Constant10/1 -> Data Store Write6/1
  Constant4/1 -> Function Caller1/3
  Constant2/1 -> Function Caller/1
  Constant7/1 -> Data Store Write1/1
  Constant9/1 -> Data Store Write4/1
  Constant6/1 -> Function Caller1/2
  Constant8/1 -> Data Store Write5/1

== system Test/Subsystem/燃油显示/Initialize Function1 ==
  Constant1 : Constant  Value=0  OutDataTypeStr=uint8
  Constant2 : Constant  Value=SIG_CLASS_HMI_TT  OutDataTypeStr=uint8
  Constant3 : Constant  Value=TT_FUEL_LEVEL_LOW  OutDataTypeStr=uint16
  Constant4 : Constant  Value=0  OutDataTypeStr=uint8
  Constant5 : Constant  Value=SIG_CLASS_HMI_SND  OutDataTypeStr=uint8
  Constant6 : Constant  Value=SND_FUEL_LEVEL_LOW  OutDataTypeStr=uint16
  Event Listener : EventListener  DisableCoverage=on  EventType=Terminate  EventName=reset
  关闭油量低报警音 : FunctionCaller  FunctionPrototype=rte_set_uint8_val(type,id,val)  InputArgumentSpecifications=uint8(1), uint16(1), uint8(1)  OutputArgumentSpecifications=<Enter example>
  熄灭油量低报警灯 : FunctionCaller  FunctionPrototype=rte_set_uint8_val(type,id,val)  InputArgumentSpecifications=uint8(1), uint16(1), uint8(1)  OutputArgumentSpecifications=<Enter example>
  wires:
  Constant1/1 -> 熄灭油量低报警灯/3
  Constant2/1 -> 熄灭油量低报警灯/1
  Constant3/1 -> 熄灭油量低报警灯/2
  Constant6/1 -> 关闭油量低报警音/2
  Constant5/1 -> 关闭油量低报警音/1
  Constant4/1 -> 关闭油量低报警音/3

== system Test/Subsystem/燃油显示/L5000车型获取油箱数据 ==
  Action Port : ActionPort
  Constant : Constant  Value=SYSSIG_LNN_MODE  OutDataTypeStr=uint16
  Constant1 : Constant  Value=SIG_CLASS_SYS  OutDataTypeStr=uint8
  LNN : Subsystem  TreatAsAtomicUnit=on
  Merge : Merge
  判断系统是否处于LNN状态 : If  IfExpression=u1 == 1
  读取系统LNN状态 : FunctionCaller  FunctionPrototype=val = rte_get_uint8_val(type,id)  InputArgumentSpecifications=uint8(1),uint16(1)  OutputArgumentSpecifications=uint8(1)
  非LNN : Subsystem  TreatAsAtomicUnit=on
  fuel_bus : Outport
  wires:
  Constant1/1 -> 读取系统LNN状态/1
  Constant/1 -> 读取系统LNN状态/2
  读取系统LNN状态/1 -> 判断系统是否处于LNN状态/1
  判断系统是否处于LNN状态/1 -> LNN/Action
  判断系统是否处于LNN状态/2 -> 非LNN/Action
  Merge/1 -> fuel_bus/1
  LNN/1(fuel_bus) -> Merge/1
  非LNN/1(fuel_bus) -> Merge/2

== system Test/Subsystem/燃油显示/其他车型获取油箱数据 ==
  Action Port : ActionPort
  Bus Creator : BusCreator  Inputs=3
  Constant : Constant  Value=0  OutDataTypeStr=uint8
  Constant1 : Constant  Value=0  OutDataTypeStr=single
  Constant2 : Constant  Value=0  OutDataTypeStr=uint8
  fuel_bus : Outport
  wires:
  Bus Creator/1 -> fuel_bus/1
  Constant1/1 -> Bus Creator/2  "percent"
  Constant/1 -> Bus Creator/1  "state"
  Constant2/1 -> Bus Creator/3  "msg"

== system Test/Subsystem/燃油显示/失效状态 ==
  In Bus Element : Inport  PortName=fuel_bus  Element=state
  Action Port : ActionPort
  判断当前信号是否有效 : If  IfExpression=u1 == 0
  无效 : Subsystem  TreatAsAtomicUnit=on
  有效 : Subsystem  TreatAsAtomicUnit=on
  wires:
  In Bus Element/1 -> 判断当前信号是否有效/1
  判断当前信号是否有效/1 -> 无效/Action
  判断当前信号是否有效/2 -> 有效/Action

== system Test/Subsystem/燃油显示/正常状态 ==
  In Bus Element : Inport  PortName=fuel_bus  Element=state
  In Bus Element1 : Inport  PortName=fuel_bus  Element=percent
  In Bus Element2 : Inport  PortName=fuel_bus  Element=msg
  Action Port : ActionPort
  Constant1 : Constant  Value=SIG_CLASS_COMTX  OutDataTypeStr=uint8
  Constant2 : Constant  Value=TXSIG_MD_OilPercent  OutDataTypeStr=uint16
  判断当前信号是否有效 : If  IfExpression=u1 == 0
  外发油量百分比 : FunctionCaller  FunctionPrototype=rte_set_uint8_val(type,id,val)  InputArgumentSpecifications=uint8(1), uint16(1), uint8(1)  OutputArgumentSpecifications=<Enter example>
  无效 : Subsystem  TreatAsAtomicUnit=on
  有效 : Subsystem  TreatAsAtomicUnit=on
  wires:
  判断当前信号是否有效/2 -> 有效/Action
  判断当前信号是否有效/1 -> 无效/Action
  In Bus Element/1 -> 判断当前信号是否有效/1
  In Bus Element1/1 -> 有效/1(fuel_percent)
  In Bus Element2/1 -> 外发油量百分比/3
  Constant2/1 -> 外发油量百分比/2
  Constant1/1 -> 外发油量百分比/1

== system Test/Subsystem/Test/Simulink Function/车型_ ==
  车型输入 : Inport  OutDataTypeStr=uint16
  Action Port : ActionPort
  Out1 : Outport  OutDataTypeStr=uint16
  wires:
  车型输入/1 -> Out1/1

== system Test/Subsystem/Test/Simulink Function/车速_ ==
  车型输入1 : Inport  OutDataTypeStr=uint16
  Action Port : ActionPort
  Out1 : Outport  OutDataTypeStr=uint16
  wires:
  车型输入1/1 -> Out1/1

== system Test/Subsystem/Test/Simulink Function1/If Action Subsystem ==
  油箱电阻 : Inport  OutDataTypeStr=uint32
  Action Port : ActionPort
  Out1 : Outport  OutDataTypeStr=uint32
  wires:
  油箱电阻/1 -> Out1/1

== system Test/Subsystem/Test/Simulink Function1/If Action Subsystem1 ==
  时间 : Inport  OutDataTypeStr=uint32
  Action Port : ActionPort
  Out1 : Outport  OutDataTypeStr=uint32
  wires:
  时间/1 -> Out1/1

== system Test/Subsystem/Test/Simulink Function2/_ ==
  in : Inport  OutDataTypeStr=uint8
  Action Port : ActionPort
  Out1 : Outport  OutDataTypeStr=uint8
  wires:
  in/1 -> Out1/1

== system Test/Subsystem/Test/Simulink Function2/车速_ ==
  in : Inport  OutDataTypeStr=uint8
  Action Port : ActionPort
  Out1 : Outport  OutDataTypeStr=uint8
  wires:
  in/1 -> Out1/1

== system Test/Subsystem/Test/Simulink Function4/CAN发_油量 ==
  车型输入 : Inport  OutDataTypeStr=uint8
  Action Port : ActionPort
  Output1 : Outport  OutDataTypeStr=uint8
  wires:
  车型输入/1 -> Output1/1

== system Test/Subsystem/Test/Simulink Function4/snd ==
  车型输入 : Inport  OutDataTypeStr=uint8
  Action Port : ActionPort
  Output : Outport  OutDataTypeStr=uint8
  wires:
  车型输入/1 -> Output/1

== system Test/Subsystem/Test/Simulink Function4/tt ==
  车型输入 : Inport  OutDataTypeStr=uint8
  Action Port : ActionPort
  Output1 : Outport  OutDataTypeStr=uint8
  wires:
  车型输入/1 -> Output1/1

== system Test/Subsystem/Test/Simulink Function4/油量显示 ==
  车型输入 : Inport  OutDataTypeStr=uint8
  Action Port : ActionPort
  Output1 : Outport  OutDataTypeStr=uint8
  wires:
  车型输入/1 -> Output1/1

== system Test/Subsystem/Test/Simulink Function4/油量真实 ==
  车型输入 : Inport  OutDataTypeStr=uint8
  Action Port : ActionPort
  Output1 : Outport  OutDataTypeStr=uint8
  wires:
  车型输入/1 -> Output1/1

== system Test/Subsystem/燃油显示/L5000车型获取油箱数据/LNN ==
  Action Port : ActionPort
  Constant : Constant  Value=RXSIG_CPD1_FuelMassSignal  OutDataTypeStr=uint16
  Constant1 : Constant  Value=SIG_CLASS_COMRX  OutDataTypeStr=uint8
  Merge : Merge
  判断CPD1油箱液位信号 是否有效 : If  NumInputs=2  IfExpression=u1 <= 250 & u2 == 1
  无效 : Subsystem  TreatAsAtomicUnit=on
  有效 : Subsystem  TreatAsAtomicUnit=on
  读取CPD1 SPN523767 信号 : FunctionCaller  FunctionPrototype=val = rte_get_uint8_val(type,id)  InputArgumentSpecifications=uint8(1),uint16(1)  OutputArgumentSpecifications=uint8(1)
  读取CPD1 SPN523767 信号状态 : FunctionCaller  FunctionPrototype=val = rte_com_get_rxsig_state(id)  InputArgumentSpecifications=uint16(1)  OutputArgumentSpecifications=uint8(1)
  fuel_bus : Outport
  wires:
  Constant/1 -> 读取CPD1 SPN523767 信号状态/1, 读取CPD1 SPN523767 信号/2
  Constant1/1 -> 读取CPD1 SPN523767 信号/1
  读取CPD1 SPN523767 信号/1 -> 有效/1(fuel_val), 判断CPD1油箱液位信号 是否有效/1
  读取CPD1 SPN523767 信号状态/1 -> 判断CPD1油箱液位信号 是否有效/2
  Merge/1 -> fuel_bus/1
  判断CPD1油箱液位信号 是否有效/1 -> 有效/Action
  判断CPD1油箱液位信号 是否有效/2 -> 无效/Action
  无效/1(fuel_bus) -> Merge/1
  有效/1(fuel_bus) -> Merge/2

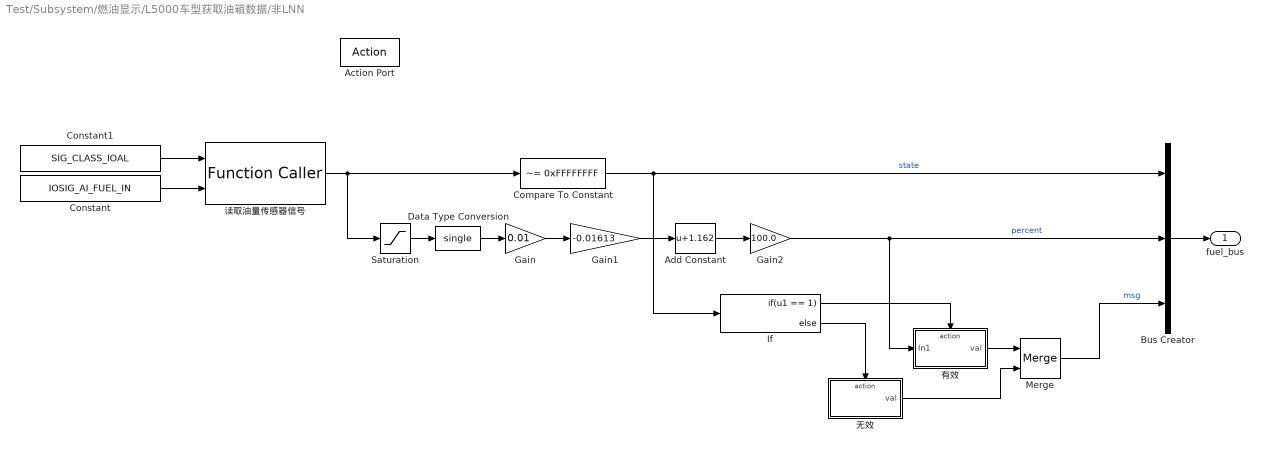
== system Test/Subsystem/燃油显示/L5000车型获取油箱数据/非LNN ==
  Action Port : ActionPort
  Add Constant : Bias  Bias=1.162
  Bus Creator : BusCreator  Inputs=3
  Compare To Constant : simulink/Logic and Bit Operations/Compare To Constant  relop=~=  const=0xFFFFFFFF  OutDataTypeStr=uint8
  Constant : Constant  Value=IOSIG_AI_FUEL_IN  OutDataTypeStr=uint16
  Constant1 : Constant  Value=SIG_CLASS_IOAL  OutDataTypeStr=uint8
  Data Type Conversion : DataTypeConversion  OutDataTypeStr=single
  Gain : Gain  Gain=0.01  ParamDataTypeStr=single  OutDataTypeStr=single  RndMeth=Round
  Gain1 : Gain  Gain=-0.01613  ParamDataTypeStr=single  OutDataTypeStr=single  RndMeth=Round
  Gain2 : Gain  Gain=100.0  ParamDataTypeStr=single  OutDataTypeStr=single  RndMeth=Round
  If : If  IfExpression=u1 == 1
  Merge : Merge
  Saturation : Saturate  UpperLimit=7200  LowerLimit=1000  OutDataTypeStr=uint32
  无效 : Subsystem  TreatAsAtomicUnit=on
  有效 : Subsystem  TreatAsAtomicUnit=on
  读取油量传感器信号 : FunctionCaller  FunctionPrototype=val = rte_get_uint32_val(type,id)  InputArgumentSpecifications=uint8(1),uint16(1)  OutputArgumentSpecifications=uint32(1)
  fuel_bus : Outport
  wires:
  Constant/1 -> 读取油量传感器信号/2
  Constant1/1 -> 读取油量传感器信号/1
  读取油量传感器信号/1 -> Compare To Constant/1, Saturation/1
  Compare To Constant/1 -> Bus Creator/1, If/1  "state"
  Bus Creator/1 -> fuel_bus/1
  Add Constant/1 -> Gain2/1
  Gain1/1 -> Add Constant/1
  Gain/1 -> Gain1/1
  Data Type Conversion/1 -> Gain/1
  Gain2/1 -> 有效/1(In1), Bus Creator/2  "percent"
  Merge/1 -> Bus Creator/3  "msg"
  If/1 -> 有效/Action
  If/2 -> 无效/Action
  有效/1(val) -> Merge/1
  无效/1(val) -> Merge/2
  Saturation/1 -> Data Type Conversion/1

== system Test/Subsystem/燃油显示/失效状态/无效 ==
  Action Port : ActionPort
  Constant : Constant  Value=0  OutDataTypeStr=uint8
  清除时间记录标志 : DataStoreWrite  DataStoreName=tnc_time_log_flag  IndexOptions=Index vector (dialog)  Indices=1  OutputSizes=1
  wires:
  Constant/1 -> 清除时间记录标志/1

== system Test/Subsystem/燃油显示/失效状态/有效 ==
  Action Port : ActionPort
  Data Store Read2 : DataStoreRead  DataStoreName=tnc_time_log_flag  IndexOptions=Index vector (dialog)  Indices=1  OutputSizes=1
  判断失效模式下是否 记录过报文有效时间 : If  IfExpression=u1 == 2
  有记录 : Subsystem  TreatAsAtomicUnit=on
  未记录 : Subsystem  TreatAsAtomicUnit=on
  wires:
  Data Store Read2/1 -> 判断失效模式下是否 记录过报文有效时间/1
  判断失效模式下是否 记录过报文有效时间/1 -> 有记录/Action
  判断失效模式下是否 记录过报文有效时间/2 -> 未记录/Action

== system Test/Subsystem/燃油显示/正常状态/无效 ==
  Action Port : ActionPort
  Data Store Read1 : DataStoreRead  DataStoreName=tnc_time_log_flag  IndexOptions=Index vector (dialog)  Indices=1  OutputSizes=1
  判断失效模式下是否 记录过报文有效时间 : If  IfExpression=u1 == 1
  有记录 : Subsystem  TreatAsAtomicUnit=on
  未记录 : Subsystem  TreatAsAtomicUnit=on
  wires:
  Data Store Read1/1 -> 判断失效模式下是否 记录过报文有效时间/1
  判断失效模式下是否 记录过报文有效时间/2 -> 未记录/Action
  判断失效模式下是否 记录过报文有效时间/1 -> 有记录/Action

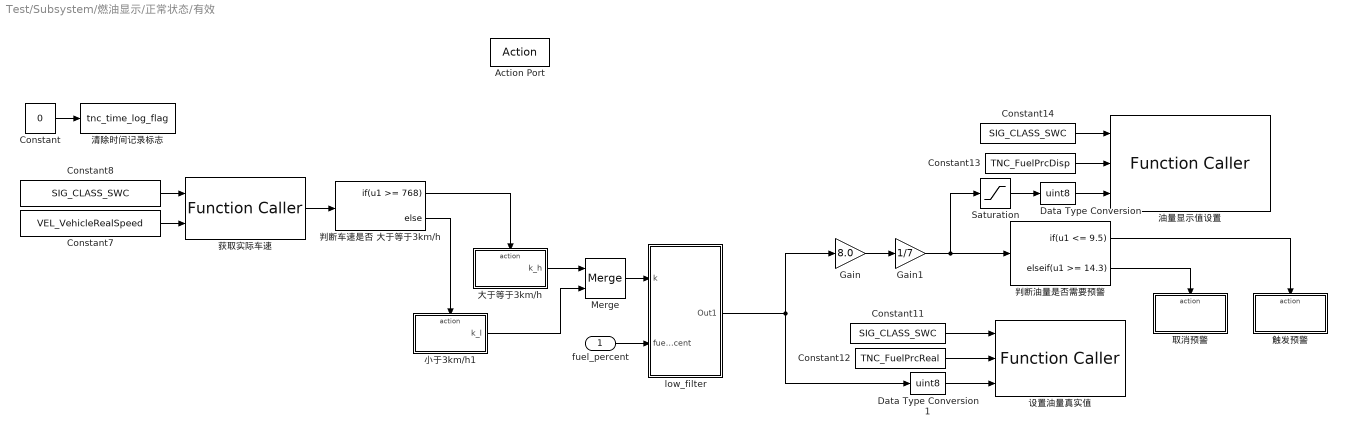
== system Test/Subsystem/燃油显示/正常状态/有效 ==
  fuel_percent : Inport  OutDataTypeStr=single
  Action Port : ActionPort
  Constant : Constant  Value=0  OutDataTypeStr=uint8
  Constant11 : Constant  Value=SIG_CLASS_SWC  OutDataTypeStr=uint8
  Constant12 : Constant  Value=TNC_FuelPrcReal  OutDataTypeStr=uint16
  Constant13 : Constant  Value=TNC_FuelPrcDisp  OutDataTypeStr=uint16
  Constant14 : Constant  Value=SIG_CLASS_SWC  OutDataTypeStr=uint8
  Constant7 : Constant  Value=VEL_VehicleRealSpeed  OutDataTypeStr=uint16
  Constant8 : Constant  Value=SIG_CLASS_SWC  OutDataTypeStr=uint8
  Data Type Conversion : DataTypeConversion  OutDataTypeStr=uint8  RndMeth=Round
  Data Type Conversion1 : DataTypeConversion  OutDataTypeStr=uint8  RndMeth=Round
  Gain : Gain  Gain=8.0  ParamDataTypeStr=single  OutDataTypeStr=single
  Gain1 : Gain  Gain=1/7  ParamDataTypeStr=single  OutDataTypeStr=single  RndMeth=Round
  Merge : Merge
  Saturation : Saturate  UpperLimit=100.0  LowerLimit=0.0  OutDataTypeStr=single  RndMeth=Round
  low_filter : Subsystem
  判断油量是否需要预警 : If  IfExpression=u1 <= 9.5  ElseIfExpressions=u1 >= 14.3  ShowElse=off
  判断车速是否 大于等于3km/h : If  IfExpression=u1 >= 768
  取消预警 : Subsystem  TreatAsAtomicUnit=on
  大于等于3km/h : Subsystem  TreatAsAtomicUnit=on
  小于3km/h1 : Subsystem  TreatAsAtomicUnit=on
  油量显示值设置 : FunctionCaller  FunctionPrototype=rte_set_uint8_val(type,id,val)  InputArgumentSpecifications=uint8(1), uint16(1), uint8(1)  OutputArgumentSpecifications=<Enter example>
  清除时间记录标志 : DataStoreWrite  DataStoreName=tnc_time_log_flag  IndexOptions=Index vector (dialog)  Indices=1  OutputSizes=1
  获取实际车速 : FunctionCaller  FunctionPrototype=val = rte_get_uint16_val(type,id)  InputArgumentSpecifications=uint8(1),uint16(1)  OutputArgumentSpecifications=uint16(1)
  触发预警 : Subsystem  TreatAsAtomicUnit=on
  设置油量真实值 : FunctionCaller  FunctionPrototype=rte_set_uint8_val(type,id,val)  InputArgumentSpecifications=uint8(1), uint16(1), uint8(1)  OutputArgumentSpecifications=<Enter example>
  wires:
  Constant/1 -> 清除时间记录标志/1
  Constant8/1 -> 获取实际车速/1
  Constant7/1 -> 获取实际车速/2
  获取实际车速/1 -> 判断车速是否 大于等于3km/h/1
  判断车速是否 大于等于3km/h/1 -> 大于等于3km/h/Action
  判断车速是否 大于等于3km/h/2 -> 小于3km/h1/Action
  大于等于3km/h/1(k_h) -> Merge/1
  Gain/1 -> Gain1/1
  Constant14/1 -> 油量显示值设置/1
  Constant11/1 -> 设置油量真实值/1
  Constant12/1 -> 设置油量真实值/2
  Constant13/1 -> 油量显示值设置/2
  判断油量是否需要预警/1 -> 触发预警/Action
  判断油量是否需要预警/2 -> 取消预警/Action
  Gain1/1 -> 判断油量是否需要预警/1, Saturation/1
  Data Type Conversion/1 -> 油量显示值设置/3
  Data Type Conversion1/1 -> 设置油量真实值/3
  小于3km/h1/1(k_l) -> Merge/2
  Merge/1 -> low_filter/1(k)
  fuel_percent/1 -> low_filter/2(fuel_percent)
  Saturation/1 -> Data Type Conversion/1
  low_filter/1(Out1) -> Data Type Conversion1/1, Gain/1

== system Test/Subsystem/燃油显示/L5000车型获取油箱数据/LNN/无效 ==
  Action Port : ActionPort
  Bus Creator : BusCreator  Inputs=3
  Constant : Constant  Value=0  OutDataTypeStr=single
  Constant1 : Constant  Value=0  OutDataTypeStr=uint8
  Constant2 : Constant  Value=255  OutDataTypeStr=uint8
  fuel_bus : Outport
  wires:
  Constant/1 -> Bus Creator/2  "percent"
  Constant1/1 -> Bus Creator/1  "state"
  Bus Creator/1 -> fuel_bus/1
  Constant2/1 -> Bus Creator/3  "msg"

== system Test/Subsystem/燃油显示/L5000车型获取油箱数据/LNN/有效 ==
  fuel_val : Inport  OutDataTypeStr=uint8
  Action Port : ActionPort
  Bus Creator : BusCreator  Inputs=3
  Constant1 : Constant  OutDataTypeStr=uint8
  Data Type Conversion : DataTypeConversion  OutDataTypeStr=single
  Gain1 : Gain  Gain=0.4  ParamDataTypeStr=single  OutDataTypeStr=single  RndMeth=Round
  fuel_bus : Outport
  wires:
  Data Type Conversion/1 -> Gain1/1
  fuel_val/1 -> Data Type Conversion/1, Bus Creator/3  "msg"
  Bus Creator/1 -> fuel_bus/1
  Gain1/1 -> Bus Creator/2  "percent"
  Constant1/1 -> Bus Creator/1  "state"

== system Test/Subsystem/燃油显示/L5000车型获取油箱数据/非LNN/无效 ==
  Action Port : ActionPort
  Constant : Constant  Value=255  OutDataTypeStr=uint8
  val : Outport  OutDataTypeStr=uint8
  wires:
  Constant/1 -> val/1

== system Test/Subsystem/燃油显示/L5000车型获取油箱数据/非LNN/有效 ==
  In1 : Inport
  Action Port : ActionPort
  Data Type Conversion : DataTypeConversion  OutDataTypeStr=uint8
  Gain3 : Gain  Gain=2.5  ParamDataTypeStr=single  OutDataTypeStr=uint8  RndMeth=Round
  val : Outport
  wires:
  In1/1 -> Gain3/1
  Data Type Conversion/1 -> val/1
  Gain3/1 -> Data Type Conversion/1

== system Test/Subsystem/燃油显示/失效状态/有效/有记录 ==
  Action Port : ActionPort
  Constant1 : Constant  Value=5  OutDataTypeStr=uint32
  Constant2 : Constant  Value=SYSSIG_TICK_COUNT  OutDataTypeStr=uint16
  Constant3 : Constant  Value=SIG_CLASS_SYS  OutDataTypeStr=uint8
  Data Store Read2 : DataStoreRead  DataStoreName=tnc_in_abn_sig_fst_time  IndexOptions=Index vector (dialog)  Indices=1  OutputSizes=1
  Subsystem : Subsystem  TreatAsAtomicUnit=on  RTWFcnName=TNC_Time_Diff
      settings: RTWFcnNameOpts=User specified
  判断是否满足时间阈值 : If  NumInputs=2  IfExpression=u1 >= u2  ShowElse=off
  满足时间阈值 : Subsystem  TreatAsAtomicUnit=on
  获取系统时间 : FunctionCaller  FunctionPrototype=val = rte_get_uint32_val(type,id)  InputArgumentSpecifications=uint8(1),uint16(1)  OutputArgumentSpecifications=uint32(1)
  wires:
  Constant2/1 -> 获取系统时间/2
  Constant3/1 -> 获取系统时间/1
  获取系统时间/1 -> Subsystem/2(now)
  Data Store Read2/1 -> Subsystem/1(his)
  Subsystem/1(time_diff) -> 判断是否满足时间阈值/1
  Constant1/1 -> 判断是否满足时间阈值/2
  判断是否满足时间阈值/1 -> 满足时间阈值/Action

== system Test/Subsystem/燃油显示/失效状态/有效/未记录 ==
  Action Port : ActionPort
  Constant : Constant  Value=2  OutDataTypeStr=uint8
  Constant2 : Constant  Value=SYSSIG_TICK_COUNT  OutDataTypeStr=uint16
  Constant3 : Constant  Value=SIG_CLASS_SYS  OutDataTypeStr=uint8
  Data Store Write1 : DataStoreWrite  DataStoreName=tnc_in_abn_sig_fst_time  IndexOptions=Index vector (dialog)  Indices=1  OutputSizes=1
  失效模式下记录过报文有效时间 : DataStoreWrite  DataStoreName=tnc_time_log_flag  IndexOptions=Index vector (dialog)  Indices=1  OutputSizes=1
  获取系统时间 : FunctionCaller  FunctionPrototype=val = rte_get_uint32_val(type,id)  InputArgumentSpecifications=uint8(1),uint16(1)  OutputArgumentSpecifications=uint32(1)
  wires:
  Constant/1 -> 失效模式下记录过报文有效时间/1
  Constant3/1 -> 获取系统时间/1
  Constant2/1 -> 获取系统时间/2
  获取系统时间/1 -> Data Store Write1/1

== system Test/Subsystem/燃油显示/正常状态/无效/有记录 ==
  Action Port : ActionPort
  Constant1 : Constant  Value=5*1000  OutDataTypeStr=uint32
  Constant2 : Constant  Value=SYSSIG_TICK_COUNT  OutDataTypeStr=uint16
  Constant3 : Constant  Value=SIG_CLASS_SYS  OutDataTypeStr=uint8
  Data Store Read2 : DataStoreRead  DataStoreName=tnc_in_nor_sig_fst_time  IndexOptions=Index vector (dialog)  Indices=1  OutputSizes=1
  Subsystem : Subsystem  TreatAsAtomicUnit=on  RTWFcnName=TNC_Time_Diff
      settings: RTWFcnNameOpts=User specified
  判断是否满足时间阈值 : If  NumInputs=2  IfExpression=u1 >= u2  ShowElse=off
  满足时间阈值 进入失效模式 时间记录标志复位 : Subsystem  TreatAsAtomicUnit=on
  获取系统时间 : FunctionCaller  FunctionPrototype=val = rte_get_uint32_val(type,id)  InputArgumentSpecifications=uint8(1),uint16(1)  OutputArgumentSpecifications=uint32(1)
  wires:
  Constant2/1 -> 获取系统时间/2
  Constant3/1 -> 获取系统时间/1
  获取系统时间/1 -> Subsystem/2(now)
  Data Store Read2/1 -> Subsystem/1(his)
  Subsystem/1(time_diff) -> 判断是否满足时间阈值/1
  Constant1/1 -> 判断是否满足时间阈值/2
  判断是否满足时间阈值/1 -> 满足时间阈值 进入失效模式 时间记录标志复位/Action

== system Test/Subsystem/燃油显示/正常状态/无效/未记录 ==
  Action Port : ActionPort
  Constant : Constant  OutDataTypeStr=uint8
  Constant2 : Constant  Value=SYSSIG_TICK_COUNT  OutDataTypeStr=uint16
  Constant3 : Constant  Value=SIG_CLASS_SYS  OutDataTypeStr=uint8
  Data Store Write1 : DataStoreWrite  DataStoreName=tnc_in_nor_sig_fst_time  IndexOptions=Index vector (dialog)  Indices=1  OutputSizes=1
  正常模式下记录过报文失效时间 : DataStoreWrite  DataStoreName=tnc_time_log_flag  IndexOptions=Index vector (dialog)  Indices=1  OutputSizes=1
  获取系统时间 : FunctionCaller  FunctionPrototype=val = rte_get_uint32_val(type,id)  InputArgumentSpecifications=uint8(1),uint16(1)  OutputArgumentSpecifications=uint32(1)
  wires:
  Constant/1 -> 正常模式下记录过报文失效时间/1
  Constant3/1 -> 获取系统时间/1
  Constant2/1 -> 获取系统时间/2
  获取系统时间/1 -> Data Store Write1/1

== system Test/Subsystem/燃油显示/正常状态/有效/low_filter ==
  note: y(t) = K*u(t) + (1-K)*y(t-1) = y(t-1) + K*[u(t)-y(t-1)]
  k : Inport  OutDataTypeStr=single
  fuel_percent : Inport  Port=2  OutDataTypeStr=single
  Add1 : Sum  Inputs=+-  AccumDataTypeStr=single  OutDataTypeStr=single  RndMeth=Round
  Add2 : Sum  AccumDataTypeStr=single  OutDataTypeStr=single  RndMeth=Round
  Product1 : Product  OutDataTypeStr=single  RndMeth=Round
  Saturation1 : Saturate  UpperLimit=100.0  LowerLimit=0.0  OutDataTypeStr=single  RndMeth=Round
  last_spd : UnitDelay  SampleTime=-1  StateName=last_spd  HasFrameUpgradeWarning=on  StateMustResolveToSignalObject=on
  Out1 : Outport  OutDataTypeStr=single
  wires:
  last_spd/1 -> Add1/2, Add2/2
  fuel_percent/1 -> Add1/1
  Add1/1 -> Product1/1
  k/1 -> Product1/2
  Product1/1 -> Add2/1
  Add2/1 -> last_spd/1, Saturation1/1
  Saturation1/1 -> Out1/1

== system Test/Subsystem/燃油显示/正常状态/有效/取消预警 ==
  Action Port : ActionPort
  Constant1 : Constant  Value=0  OutDataTypeStr=uint8
  Constant2 : Constant  Value=SIG_CLASS_HMI_SND  OutDataTypeStr=uint8
  Constant3 : Constant  Value=SND_FUEL_LEVEL_LOW  OutDataTypeStr=uint16
  Constant4 : Constant  Value=0  OutDataTypeStr=uint8
  Constant5 : Constant  Value=SIG_CLASS_HMI_TT  OutDataTypeStr=uint8
  Constant6 : Constant  Value=TT_FUEL_LEVEL_LOW  OutDataTypeStr=uint16
  油量报警蜂鸣器关闭 : FunctionCaller  FunctionPrototype=rte_set_uint8_val(type,id,val)  InputArgumentSpecifications=uint8(1), uint16(1), uint8(1)  OutputArgumentSpecifications=<Enter example>
  燃油低报警灯关闭 : FunctionCaller  FunctionPrototype=rte_set_uint8_val(type,id,val)  InputArgumentSpecifications=uint8(1), uint16(1), uint8(1)  OutputArgumentSpecifications=<Enter example>
  wires:
  Constant5/1 -> 燃油低报警灯关闭/1
  Constant4/1 -> 燃油低报警灯关闭/3
  Constant6/1 -> 燃油低报警灯关闭/2
  Constant3/1 -> 油量报警蜂鸣器关闭/2
  Constant1/1 -> 油量报警蜂鸣器关闭/3
  Constant2/1 -> 油量报警蜂鸣器关闭/1

== system Test/Subsystem/燃油显示/正常状态/有效/大于等于3km//h ==
  Action Port : ActionPort
  Constant : Constant  Value=0.01  OutDataTypeStr=single
  filter_higher_3 : MATLAB Function  Commented=on  TreatAsAtomicUnit=on
  k_h : Outport  OutDataTypeStr=single
  wires:
  Constant/1 -> k_h/1

== system Test/Subsystem/燃油显示/正常状态/有效/小于3km//h1 ==
  Action Port : ActionPort
  Constant : Constant  Value=0.3  OutDataTypeStr=single
  filter_lower_3 : MATLAB Function  Commented=on  TreatAsAtomicUnit=on
  k_l : Outport  OutDataTypeStr=single
  wires:
  Constant/1 -> k_l/1

== system Test/Subsystem/燃油显示/正常状态/有效/触发预警 ==
  Action Port : ActionPort
  Constant1 : Constant  OutDataTypeStr=uint8
  Constant2 : Constant  Value=SIG_CLASS_HMI_SND  OutDataTypeStr=uint8
  Constant3 : Constant  Value=SND_FUEL_LEVEL_LOW  OutDataTypeStr=uint16
  Constant4 : Constant  OutDataTypeStr=uint8
  Constant5 : Constant  Value=SIG_CLASS_HMI_TT  OutDataTypeStr=uint8
  Constant6 : Constant  Value=TT_FUEL_LEVEL_LOW  OutDataTypeStr=uint16
  油量报警蜂鸣器鸣叫 : FunctionCaller  FunctionPrototype=rte_set_uint8_val(type,id,val)  InputArgumentSpecifications=uint8(1), uint16(1), uint8(1)  OutputArgumentSpecifications=<Enter example>
  燃油低报警灯长亮 : FunctionCaller  FunctionPrototype=rte_set_uint8_val(type,id,val)  InputArgumentSpecifications=uint8(1), uint16(1), uint8(1)  OutputArgumentSpecifications=<Enter example>
  wires:
  Constant5/1 -> 燃油低报警灯长亮/1
  Constant4/1 -> 燃油低报警灯长亮/3
  Constant6/1 -> 燃油低报警灯长亮/2
  Constant3/1 -> 油量报警蜂鸣器鸣叫/2
  Constant1/1 -> 油量报警蜂鸣器鸣叫/3
  Constant2/1 -> 油量报警蜂鸣器鸣叫/1

== system Test/Subsystem/燃油显示/失效状态/有效/有记录/Subsystem ==
  his : Inport  OutDataTypeStr=uint32
  now : Inport  Port=2  OutDataTypeStr=uint32
  If : If  NumInputs=2  IfExpression=u1 > u2  ElseIfExpressions=u1 < u2
  Merge : Merge  Inputs=3
  历史值大于当前值 : Subsystem  TreatAsAtomicUnit=on
  历史值小于当前值 : Subsystem  TreatAsAtomicUnit=on
  历史值等于当前值 : Subsystem  TreatAsAtomicUnit=on
  time_diff : Outport  OutDataTypeStr=uint32
  wires:
  his/1 -> 历史值小于当前值/1(his), 历史值大于当前值/1(his), If/1
  now/1 -> 历史值小于当前值/2(now), 历史值大于当前值/2(now), If/2
  If/1 -> 历史值大于当前值/Action
  If/2 -> 历史值小于当前值/Action
  If/3 -> 历史值等于当前值/Action
  历史值大于当前值/1(time_diff) -> Merge/1
  历史值小于当前值/1(time_diff) -> Merge/2
  历史值等于当前值/1(time_diff) -> Merge/3
  Merge/1 -> time_diff/1
